simulink library "c_slow_lib"  (R2017a)
settings: Solver=VariableStepAuto  StartTime=0.0  StopTime=10.0  RelTol=1e-3
settings Model: Creator=cyarp  LastModifiedBy=cyarp

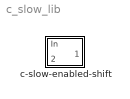
== system c_slow_lib ==
  c-slow-enabled-shift : Subsystem  mask(CSlowEnabledShift){ShareFactor=1}
      mask prompts: ShareFactor "Share Factor"
      mask help: Provides a shift register that is capable of retaining state. Used for c-slow resource sharing.

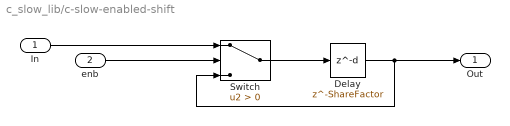
== system c_slow_lib/c-slow-enabled-shift ==
  In : Inport
  enb : Inport  Port=2  OutDataTypeStr=boolean
  Delay : Delay  DelayLength=ShareFactor  InitialCondition=0
  Switch : Switch  Criteria=u2 > Threshold
  Out : Outport
  wires:
  Switch/1 -> Delay/1
  enb/1 -> Switch/2
  In/1 -> Switch/1
  Delay/1 -> Out/1, Switch/3
